simulink model "controller_sh_arduino"  (R2021b)
settings: Solver=FixedStepAuto  StartTime=0.0  StopTime=10.0  FixedStep=0.001  RelTol=1e-3  EnableMultiTasking=on
libraries: arduinolib x7, simulink x2
settings Model: ExtModeTrigDuration=2  Creator=Gaia  LastModifiedBy=sagai
settings OptimizationCC: EnhancedBackFolding=on  PassReuseOutputArgsAs=Individual arguments  ZeroExternalMemoryAtStartup=off  ZeroInternalMemoryAtStartup=off  MaxStackSize=64  OptimizeBlockOrder=speed  DifferentSizesBufferReuse=on  OptimizationCustomize=off  EfficientTunableParamExpr=on
settings DebuggingCC: ParameterTunabilityLossMsg=error
settings HardwareCC: ProdBitPerInt=16  ProdBitPerPointer=16  ProdBitPerSizeT=16  ProdBitPerPtrDiffT=16  ProdLargestAtomicFloat=None  ProdWordSize=8  ProdHWDeviceType=Atmel->AVR
settings SFSimCC: MATLABDynamicMemAlloc=off
settings RTWCC: Description=Embedded Coder  SystemTargetFile=ert.tlc  HardwareBoard=Arduino Uno  TemplateMakefile=ert_default_tmf  Toolchain=Arduino AVR  BuildConfiguration=Faster Runs  IncludeHyperlinkInReport=on
settings CodeAppCC: ForceParamTrailComments=on  IgnoreCustomStorageClasses=off  OperatorAnnotations=on  SimulinkDataObjDesc=on  SFDataObjDesc=on  InsertBlockDesc=on
settings ERTTargetCC: SupportContinuousTime=on  SupportNonInlinedSFcns=on  SupportVariableSizeSignals=on  ExtModeTransport=3  ExtModeStaticAlloc=on  ExtModeStaticAllocSize=250  ExtModeMexFile=ext_xcp  ExtModeIntrfLevel=Level2 - Open

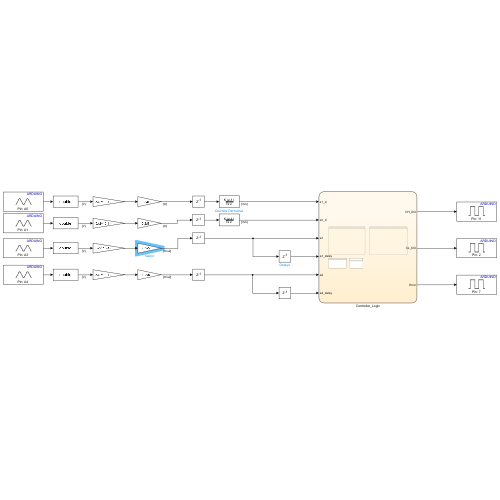
[thumbnail: Simulink's stored preview of the top-level diagram]
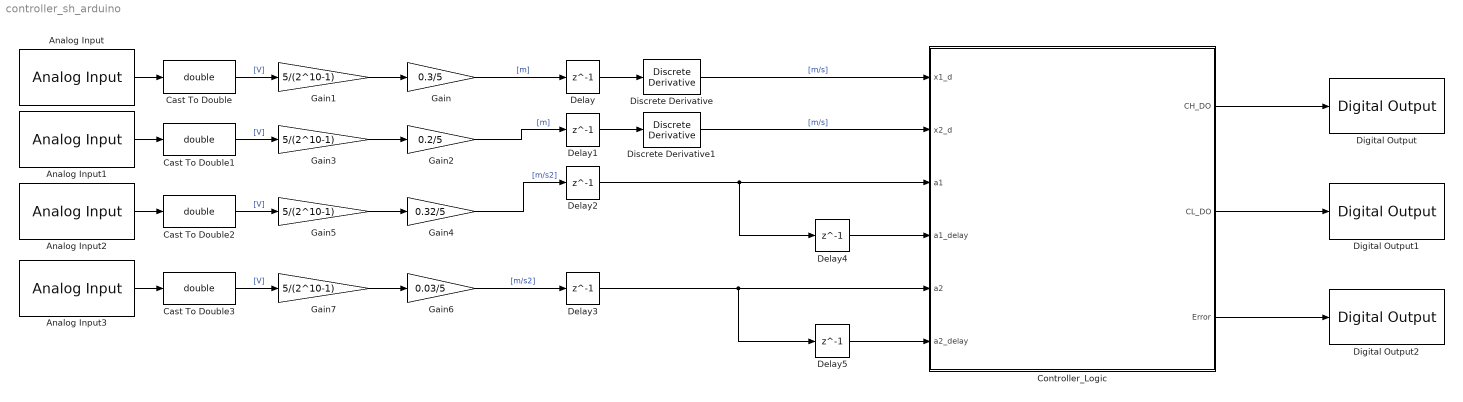
== system controller_sh_arduino ==
  Analog Input : arduinolib/Analog Input  pinNumber=0  ReadResultsOnly=off  ConversionTriggerSource=Software  ExternalTriggerType=uint32( 0 )  OutputDataType=uint16  EnableConversionCompleteNotify=off  EnableOuputStatus=off  SampleTime=-1  blockPlatform=arduino
  Analog Input1 : arduinolib/Analog Input  pinNumber=1  ReadResultsOnly=off  ConversionTriggerSource=Software  ExternalTriggerType=uint32( 0 )  OutputDataType=uint16  EnableConversionCompleteNotify=off  EnableOuputStatus=off  SampleTime=-1  blockPlatform=arduino
  Analog Input2 : arduinolib/Analog Input  pinNumber=3  ReadResultsOnly=off  ConversionTriggerSource=Software  ExternalTriggerType=uint32( 0 )  OutputDataType=uint16  EnableConversionCompleteNotify=off  EnableOuputStatus=off  SampleTime=-1  blockPlatform=arduino
  Analog Input3 : arduinolib/Analog Input  pinNumber=4  ReadResultsOnly=off  ConversionTriggerSource=Software  ExternalTriggerType=uint32( 0 )  OutputDataType=uint16  EnableConversionCompleteNotify=off  EnableOuputStatus=off  SampleTime=-1  blockPlatform=arduino
  Cast To Double{,1..3} (4 alike) : DataTypeConversion  OutDataTypeStr=double
  Controller_Logic : Stateflow chart  TreatAsAtomicUnit=on
      settings: PortSchema="{\"entries\":[{\"content\":{\"sides\":[{\"content\":{\"connectorIds\":[\"In1\",\"In2\",\"In5\",\"In3\",\"In6\",\"In4\"]},\"type\":\"ConnectorPlacement.EquallySpacedRectSide\",\"uuid\":\"03fcdeea-861d-403d-a713-017c2a853cd0\"},{\"content\":{\"connectorIds\":[\"Out1\",\"Out2\",\"Out3\"],\"side\":\"RIGHT\"},\"type\":\"ConnectorPlacement.EquallySpacedRectSide\",\"uuid\":\"c533f712-70b6-4dd9-9569-6aad03cb8087\"},{\"content\":{\"connectorIds\":[],\"side\":\"TOP\"},\"type\":\"ConnectorPlacement.EquallySpacedRectSide\",\"uuid\":\"58c96a87-d27c-4904-8775-afc8acbd3a66\"}]},\"type\":\"ConnectorPlacement.EquallySpacedConnector\",\"uuid\":\"db3d0038-3e4d-416e-9575-e84c800f913b\"}],\"packageUris\":[\"http://schema.mathworks.com/mf0/Connector/R2020b\"],\"version\":\"1.0\"}"
  Delay{,1..5} (6 alike) : Delay  DelayLength=1  InitialCondition=0
  Digital Output : arduinolib/Digital Output  pinNumber=11  Direction=output  blockPlatform=arduino
  Digital Output1 : arduinolib/Digital Output  pinNumber=2  Direction=output  blockPlatform=arduino
  Digital Output2 : arduinolib/Digital Output  pinNumber=7  Direction=output  blockPlatform=arduino
  Discrete Derivative : simulink/Discrete/Discrete Derivative  gainval=1.0  ICPrevScaledInput=0.0  OutMin=[]  OutMax=[]  OutDataType=fixdt(1, 16)  OutScaling=2^-10  DoSatur=off
  Discrete Derivative1 : simulink/Discrete/Discrete Derivative  gainval=1.0  ICPrevScaledInput=0.0  OutMin=[]  OutMax=[]  OutDataType=fixdt(1, 16)  OutScaling=2^-10  DoSatur=off
  Gain : Gain  Gain=0.3/5
  Gain{1,3,5,7} (4 alike) : Gain  Gain=5/(2^10-1)
  Gain2 : Gain  Gain=0.2/5
  Gain4 : Gain  Gain=0.32/5
  Gain6 : Gain  Gain=0.03/5
  wires:
  Controller_Logic/1(CH_DO) -> Digital Output/1
  Controller_Logic/2(CL_DO) -> Digital Output1/1
  Controller_Logic/3(Error) -> Digital Output2/1
  Analog Input/1 -> Cast To Double/1
  Cast To Double/1 -> Gain1/1  "[V]"
  Gain1/1 -> Gain/1
  Cast To Double1/1 -> Gain3/1  "[V]"
  Gain3/1 -> Gain2/1
  Analog Input1/1 -> Cast To Double1/1
  Discrete Derivative1/1 -> Controller_Logic/2(x2_d)  "[m/s]"
  Delay1/1 -> Discrete Derivative1/1
  Delay3/1 -> Controller_Logic/6(a2), Delay5/1
  Delay2/1 -> Delay4/1, Controller_Logic/5(a1)
  Discrete Derivative/1 -> Controller_Logic/1(x1_d)  "[m/s]"
  Gain/1 -> Delay/1  "[m]"
  Delay/1 -> Discrete Derivative/1
  Gain2/1 -> Delay1/1  "[m]"
  Delay4/1 -> Controller_Logic/3(a1_delay)
  Delay5/1 -> Controller_Logic/4(a2_delay)
  Gain5/1 -> Gain4/1
  Cast To Double2/1 -> Gain5/1  "[V]"
  Gain7/1 -> Gain6/1
  Cast To Double3/1 -> Gain7/1  "[V]"
  Analog Input2/1 -> Cast To Double2/1
  Analog Input3/1 -> Cast To Double3/1
  Gain4/1 -> Delay2/1  "[m/s2]"
  Gain6/1 -> Delay3/1  "[m/s2]"

== stateflow chart controller_sh_arduino/Controller_Logic ==
  state On_Off_Logic [parallel]
    settings: executionOrder=1
    state OFF
      en:
      CH_DO = 1;
      CL_DO = 0;
    state ON
      during: XTable(x1_d,x2_d)
    (default) -> OFF
    OFF -> ON : [Safe_State==0]
    ON -> OFF : [Safe_State==1]
  state Error_Logic [parallel]
    settings: executionOrder=2
    state OK
      en:
      Error = 0;
      Safe_State= 0;
    state ERROR
      en:
      Error = 1;
      Safe_State=1;
    (default) -> OK
    OK -> ERROR : [duration(NotChange(a1, a1_delay),msec)>=20 || duration(NotChange(a2, a2_delay),msec)>=20]
  data: v1 function_input double; v2 function_input double; a_now function_input double; a_after function_input double; f function_output double; CH_DO output boolean; CL_DO output boolean; x1_d input double; x2_d input double; Error output boolean; Safe_State local double; a1_delay input double size=1; a2_delay input double size=1; a1 input double size=1; a2 input double size=1
  function XTable(v1,v2):
    | function XTable(v1,v2)
    | 
    | aVarTruthTableCondition_1 = false;
    | aVarTruthTableCondition_2 = false;
    | 
    | 
    | % More comfort is given to the driver by switching the softer damping factor.
    | 
    | aVarTruthTableCondition_1 = logical((v1 - v2) * v1< 0);
    | 
    | % More reactivity is given to the driver by switching the harder damping factor.
    | 
    | aVarTruthTableCondition_2 = logical((v1 - v2) * v1 >= 0);
    | 
    | if (aVarTruthTableCondition_1 && ~aVarTruthTableCondition_2)
    |     A2();
    | elseif (~aVarTruthTableCondition_1 && aVarTruthTableCondition_2)
    |     A1();
    | else % Default
    |     A1();
    | end
    | 
    | function A1()
    | 
    | % Switch to harder damping factor
    | 
    | CH_DO = true;CL_DO = false;
    | 
    | function A2()
    | 
    | % Switch to softer damping factor
    | 
    | CH_DO = false;CL_DO = true;
  function f=NotChange(a_now, a_after):
    | function f=NotChange(a_now, a_after)
    |     if abs(a_now-a_after)< 1e-5 
    |         f=1;
    |     else
    |         f=0;
    |     end
    | end
